simulink model "simulink_model_vorlage"  (Simulink 7.9)
settings: Solver=ode45  StartTime=0.0  StopTime=8*pi  MaxStep=0.01  RelTol=1e-3
values from neighbouring files (symbols this model uses):
  k1 = params(1)    [ode45_dgl1n.m]    (also in ode45_script.m = -0.1; simulink_script.m = -0.1)
  k2 = params(2)    [ode45_dgl1n.m]    (also in ode45_script.m = 4; simulink_script.m = 4)
  k3 = params(3)    [ode45_dgl1n.m]    (also in ode45_script.m = 0.8; simulink_script.m = 0.8)
  k4 = params(4)    [ode45_dgl1n.m]    (also in ode45_script.m = 20; simulink_script.m = 20)
settings Model: Creator=s67707  LastModifiedBy=s67707

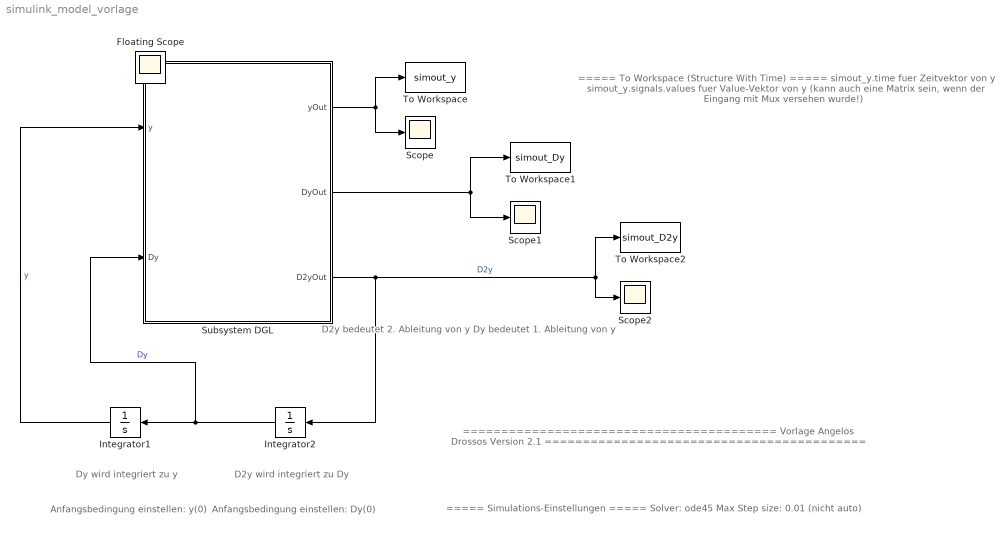
== system simulink_model_vorlage ==
  note: ===== To Workspace (Structure With Time) =====
      |
      | simout_y.time                fuer Zeitvektor von y
      | simout_y.signals.values      fuer Value-Vektor von y
      |                                                   (kann auch eine Matrix sein,
      |                                                                            wenn der Eingang mit Mux versehen wurde!)
  note: D2y wird integriert zu Dy
  note: Anfangsbedingung einstellen:
      | Dy(0)
  note: Anfangsbedingung einstellen:
      | y(0)
  note: Dy wird integriert zu y
  note: =========================================
      | Vorlage
      | Angelos Drossos
      | Version 2.1
      | ==========================================
  note: D2y bedeutet 2. Ableitung von y
      | Dy   bedeutet 1. Ableitung von y
  note: ===== Simulations-Einstellungen =====
      | Solver: ode45
      | Max Step size: 0.01 (nicht auto)
  Integrator1 : Integrator  InitialCondition=-pi/2
  Integrator2 : Integrator  InitialCondition=pi/4
  Scope : Scope
  Scope1 : Scope
      settings: SaveName=ScopeData2
  Scope2 : Scope
      settings: SaveName=ScopeData3
  Subsystem DGL : Subsystem
  To Workspace : ToWorkspace  VariableName=simout_y  SampleTime=-1  SaveFormat=Structure With Time
  To Workspace1 : ToWorkspace  VariableName=simout_Dy  SampleTime=-1  SaveFormat=Structure With Time
  To Workspace2 : ToWorkspace  VariableName=simout_D2y  SampleTime=-1  SaveFormat=Structure With Time
  Floating Scope : Scope
      settings: Floating=on
  wires:
  Subsystem DGL/3(D2yOut) -> Integrator2/1, Scope2/1, To Workspace2/1  "D2y"
  Integrator2/1 -> Integrator1/1, Subsystem DGL/2(Dy)  "Dy"
  Integrator1/1 -> Subsystem DGL/1(y)  "y"
  Subsystem DGL/1(yOut) -> Scope/1, To Workspace/1
  Subsystem DGL/2(DyOut) -> To Workspace1/1, Scope1/1

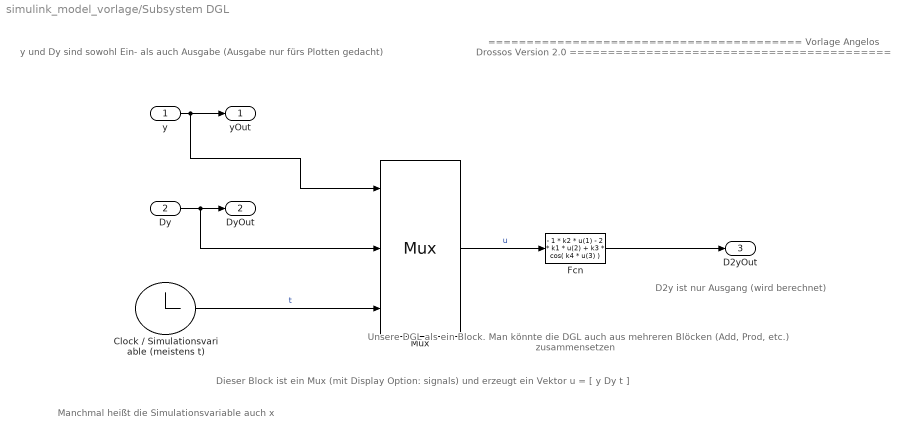
== system simulink_model_vorlage/Subsystem DGL ==
  note: y und Dy sind
      | sowohl Ein- als auch Ausgabe
      | (Ausgabe nur fürs Plotten gedacht)
  note: D2y ist nur Ausgang
      | (wird berechnet)
  note: Manchmal heißt
      | die Simulationsvariable
      | auch x
  note: Dieser Block ist ein Mux
      | (mit Display Option: signals)
      | und erzeugt ein Vektor
      | u = [ y   Dy   t ]
  note: Unsere DGL als ein Block.
      | Man könnte die DGL auch
      | aus mehreren Blöcken
      | (Add, Prod, etc.)
      | zusammensetzen
  note: =========================================
      | Vorlage
      | Angelos Drossos
      | Version 2.0
      | ==========================================
  y : Inport
  Dy : Inport  Port=2
  Clock / Simulationsvariable (meistens t) : Clock
  Fcn : Fcn  Expr=- 1 * k2 * u(1) - 2 * k1 * u(2) + k3 * cos( k4 * u(3) )
  Mux : Mux  Inputs=3
      settings: DisplayOption=signals
  yOut : Outport
  DyOut : Outport  Port=2
  D2yOut : Outport  Port=3
  wires:
  y/1 -> yOut/1, Mux/1
  Mux/1 -> Fcn/1  "u"
  Clock / Simulationsvariable (meistens t)/1 -> Mux/3  "t"
  Fcn/1 -> D2yOut/1
  Dy/1 -> Mux/2, DyOut/1
